simulink library "Command"  (R2014b)
settings: Solver=ode45  StartTime=0.0  StopTime=10.0  RelTol=1e-3
undefined symbols (not defined in the file): ConfParam
libraries: AdvancedMux x4, AdvancedDemux x1, EarthAndTargetPointing x1, EarthPointing x1, InertialAndTargetPointing x1, InertialPointing x1
settings Model: Creator=Hp  LastModifiedBy=Hp

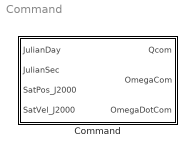
== system Command ==
  Command : Subsystem

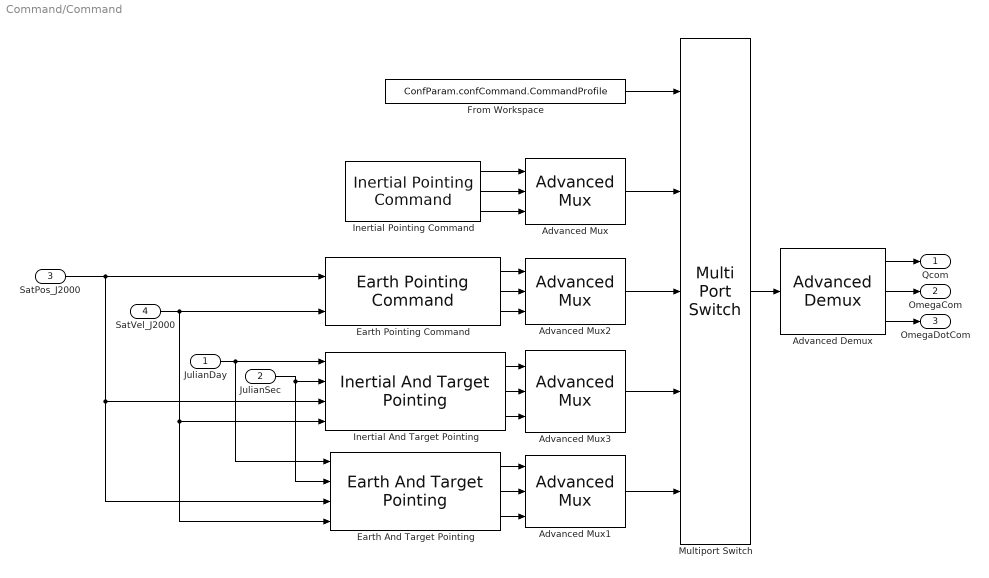
== system Command/Command ==
  JulianDay : Inport
  JulianSec : Inport  Port=2
  SatPos_J2000 : Inport  Port=3
  SatVel_J2000 : Inport  Port=4
  Advanced Demux : AdvancedDemux/Advanced Demux
  Advanced Mux{,1..3} (4 alike) : AdvancedMux/Advanced Mux
  Earth And Target Pointing : EarthAndTargetPointing/Earth And Target Pointing
  "Earth Pointing Command " : EarthPointing/Earth Pointing Command
  From Workspace : FromWorkspace  VariableName=ConfParam.confCommand.CommandProfile  SampleTime=0  Interpolate=off  OutputAfterFinalValue=Holding final value
  "Inertial And Target Pointing " : InertialAndTargetPointing/Inertial And Target Pointing 
  Inertial Pointing Command : InertialPointing/Inertial Pointing Command
  Multiport Switch : MultiPortSwitch  Inputs=4  SampleTime=ConfParam.confOrbit.dt
  Qcom : Outport
  OmegaCom : Outport  Port=2
  OmegaDotCom : Outport  Port=3
  wires:
  Multiport Switch/1 -> Advanced Demux/1
  "Earth Pointing Command "/3 -> Advanced Mux2/3
  Inertial Pointing Command/2 -> Advanced Mux/2
  Advanced Mux2/1 -> Multiport Switch/3
  Advanced Demux/3 -> OmegaDotCom/1
  Inertial Pointing Command/3 -> Advanced Mux/3
  JulianDay/1 -> Earth And Target Pointing/1, "Inertial And Target Pointing "/1
  From Workspace/1 -> Multiport Switch/1
  Advanced Demux/1 -> Qcom/1
  SatVel_J2000/1 -> "Earth Pointing Command "/2, Earth And Target Pointing/4, "Inertial And Target Pointing "/4
  SatPos_J2000/1 -> Earth And Target Pointing/3, "Inertial And Target Pointing "/3, "Earth Pointing Command "/1
  JulianSec/1 -> Earth And Target Pointing/2, "Inertial And Target Pointing "/2
  Advanced Demux/2 -> OmegaCom/1
  "Earth Pointing Command "/1 -> Advanced Mux2/1
  Advanced Mux/1 -> Multiport Switch/2
  "Earth Pointing Command "/2 -> Advanced Mux2/2
  "Inertial And Target Pointing "/3 -> Advanced Mux3/3
  Advanced Mux3/1 -> Multiport Switch/4
  "Inertial And Target Pointing "/2 -> Advanced Mux3/2
  Earth And Target Pointing/2 -> Advanced Mux1/2
  Inertial Pointing Command/1 -> Advanced Mux/1
  "Inertial And Target Pointing "/1 -> Advanced Mux3/1
  Earth And Target Pointing/3 -> Advanced Mux1/3
  Earth And Target Pointing/1 -> Advanced Mux1/1
  Advanced Mux1/1 -> Multiport Switch/5
